simulink model "model_VS_PSH"  (R2020b)
settings: Solver=ode1  StartTime=0.0  StopTime=60  RelTol=1e-3
InitFcn:
  | xInitial = init_power_wind_dfig_det;
  | %Ts=5e-6;
values from neighbouring files (symbols this model uses):
  Cap_DClink = 20000e-6    (= 0.02)    [MAIN_VS_PSH.m]
  Efficiency = 0.9    [MAIN_VS_PSH.m]
  Fnom = 60    [MAIN_VS_PSH.m]
  H = 2.7    [MAIN_VS_PSH.m]
  Initial_Head = 1    [MAIN_VS_PSH.m]
  Initial_SOC = 0.8    [MAIN_VS_PSH.m]
  kmVdc = 20e3    (= 20000)    [MAIN_VS_PSH.m]
  Kp = 1    [MAIN_VS_PSH.m]
  kp_pll = 0.236583    [MAIN_T_PSH_IEEE39.m]    (also in MAIN_VS_PSH.m)
  Kpg = 1.3466e-5    (= 1.3466e-05)    [MAIN_VS_PSH.m]
  Kpr = 4.559e-5    (= 4.559e-05)    [MAIN_VS_PSH.m]
  Kvp = 6.1584    [MAIN_VS_PSH.m]
  Lm = Lb*Lmpu    [MAIN_VS_PSH.m]
  Lph = 3e-4    (= 0.0003)    [MAIN_VS_PSH.m]
  Lr = Lb*Lrpu    [MAIN_VS_PSH.m]
  Lrleakpu = 0.11    [MAIN_VS_PSH.m]
  Ls = Lb*Lspu    [MAIN_VS_PSH.m]
  Lsleakpu = 0.102    [MAIN_VS_PSH.m]
  Max_discharge_hrs = 10    [MAIN_VS_PSH.m]
  Mode = 0    [MAIN_FS_PSH_IEEE39.m]    (also in MAIN_VS_PSH.m = 1; plots_FS_PSH_IEEE39.m = 1; plots_VS_PSH.m = 1)
  Pnom = Srated*1e6    (= 300000000)    [MAIN_VS_PSH.m]
  Pref = 0.9    [MAIN_T_PSH_IEEE39.m]    (also in MAIN_VS_PSH.m = 1)
  QnL = 0    [MAIN_VS_PSH.m]
  Qref = 0    [MAIN_VS_PSH.m]
  Rrpu = 0.00607    [MAIN_VS_PSH.m]
  Rspu = 0.0054    [MAIN_VS_PSH.m]
  sigma = 1- Lmpu*Lmpu/(Lrpu^2)    (= 0.0485899542692)    [MAIN_VS_PSH.m]
  Srated = 300    [MAIN_VS_PSH.m]
  t_sw_off = 220    [MAIN_FS_PSH_IEEE39.m]    (also in MAIN_T_PSH_IEEE39.m; MAIN_VS_PSH.m = 45)
  t_sw_on = 130    [MAIN_FS_PSH_IEEE39.m]    (also in MAIN_T_PSH_IEEE39.m; MAIN_VS_PSH.m = 35)
  Ti = 0.01    [MAIN_VS_PSH.m]
  ti_pll = 0.0224242    [MAIN_T_PSH_IEEE39.m]    (also in MAIN_VS_PSH.m)
  Tig = 59.0944    [MAIN_VS_PSH.m]
  Tir = 197.953    [MAIN_VS_PSH.m]
  Ts = 25e-6    (= 2.5e-05)    [MAIN_FS_PSH_IEEE39.m]    (also in MAIN_T_PSH_IEEE39.m; MAIN_VS_PSH.m = 1e-07)
  TurnsRatio = 0.37912    [MAIN_VS_PSH.m]
  Tvi = 0.0013532    [MAIN_VS_PSH.m]
  V1 = sqrt(2)*Vnom_grid/sqrt(3)    [MAIN_VS_PSH.m]
  Vdc_ref = 40e3    (= 40000)    [MAIN_VS_PSH.m]
  Vnom_grid = 18e3    (= 18000)    [MAIN_VS_PSH.m]
  W1 = 2*pi*Fnom    (= 376.991118431)    [MAIN_VS_PSH.m]
  Xph = Lph*W1    (= 0.113097335529)    [MAIN_VS_PSH.m]
undefined symbols (not defined in the file or in its folder): magnitude
libraries: powerlib x49, powerlib_meascontrol x21, pid_lib x10, simulink_extras x4, simulink x1
(part 2 of 3)

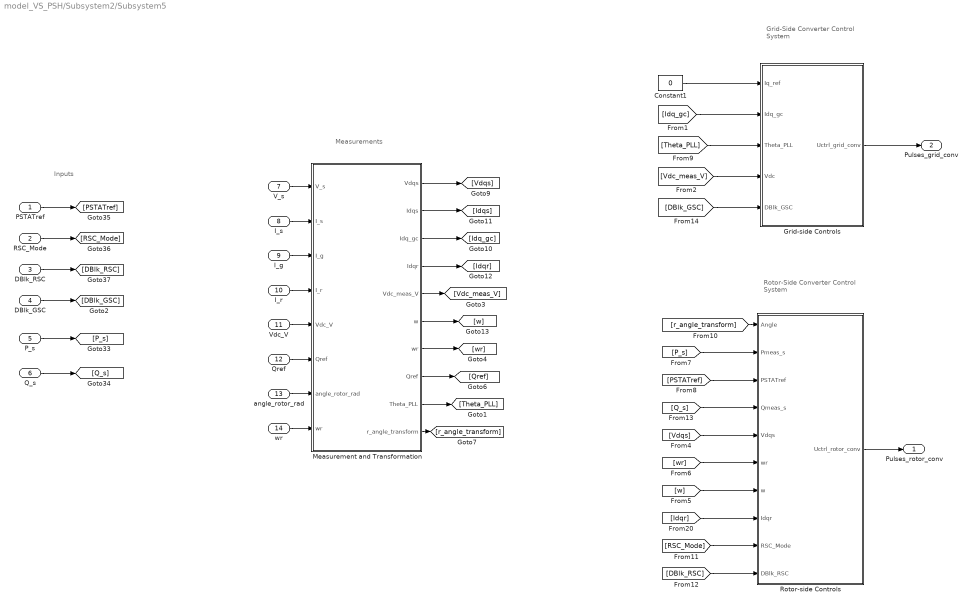
== system model_VS_PSH/Subsystem2/Subsystem5 ==
  note: Measurements
  note: Inputs
  note: Grid-Side Converter
      | Control System
  note: Rotor-Side Converter
      | Control System
  PSTATref : Inport
  RSC_Mode : Inport  Port=2
  DBlk_RSC : Inport  Port=3
  DBlk_GSC : Inport  Port=4
  P_s : Inport  Port=5
  Q_s : Inport  Port=6
  V_s : Inport  Port=7
  I_s : Inport  Port=8
  I_g : Inport  Port=9
  I_r : Inport  Port=10
  Vdc_V : Inport  Port=11
  Qref : Inport  Port=12
  angle_rotor_rad : Inport  Port=13
  wr : Inport  Port=14
  Constant1 : Constant  Value=0
  Grid-side Controls : Subsystem
  Measurement and Transformation : Subsystem
  Rotor-side Controls : Subsystem
  Pulses_rotor_conv : Outport  VectorParamsAs1DForOutWhenUnconnected=off
  Pulses_grid_conv : Outport  Port=2  VectorParamsAs1DForOutWhenUnconnected=off
  wires:
  PSTATref/1 -> [PSTATref]
  Q_s/1 -> [Q_s]
  P_s/1 -> [P_s]
  RSC_Mode/1 -> [RSC_Mode]
  DBlk_GSC/1 -> [DBlk_GSC]
  DBlk_RSC/1 -> [DBlk_RSC]
  Measurement and Transformation/7("wr ") -> [wr]
  Qref/1 -> Measurement and Transformation/6(Qref)
  wr/1 -> Measurement and Transformation/8(wr)
  Measurement and Transformation/5(Vdc_meas_V) -> [Vdc_meas_V]
  V_s/1 -> Measurement and Transformation/1(V_s)
  I_g/1 -> Measurement and Transformation/3(I_g)
  I_s/1 -> Measurement and Transformation/2(I_s)
  Measurement and Transformation/3(Idq_gc) -> [Idq_gc]
  Measurement and Transformation/4(Idqr) -> [Idqr]
  angle_rotor_rad/1 -> Measurement and Transformation/7(angle_rotor_rad)
  Measurement and Transformation/8("Qref ") -> [Qref]
  Measurement and Transformation/9(Theta_PLL) -> [Theta_PLL]
  Measurement and Transformation/1(Vdqs) -> [Vdqs]
  Measurement and Transformation/10(r_angle_transform) -> [r_angle_transform]
  Measurement and Transformation/2(Idqs) -> [Idqs]
  Measurement and Transformation/6(w) -> [w]
  Vdc_V/1 -> Measurement and Transformation/5(Vdc_V)
  I_r/1 -> Measurement and Transformation/4(I_r)
  Rotor-side Controls/1(Uctrl_rotor_conv) -> Pulses_rotor_conv/1
  [P_s] -> Rotor-side Controls/2(Pmeas_s)
  [DBlk_GSC] -> Grid-side Controls/5(DBlk_GSC)
  Grid-side Controls/1(Uctrl_grid_conv) -> Pulses_grid_conv/1
  [RSC_Mode] -> Rotor-side Controls/9(RSC_Mode)
  [PSTATref] -> Rotor-side Controls/3(PSTATref)
  [wr] -> Rotor-side Controls/6(wr)
  [DBlk_RSC] -> Rotor-side Controls/10(DBlk_RSC)
  [Idqr] -> Rotor-side Controls/8(Idqr)
  [r_angle_transform] -> Rotor-side Controls/1(Angle)
  [Idq_gc] -> Grid-side Controls/2(Idq_gc)
  [Vdqs] -> Rotor-side Controls/5(Vdqs)
  [Theta_PLL] -> Grid-side Controls/3(Theta_PLL)
  Constant1/1 -> Grid-side Controls/1(Iq_ref)
  [Q_s] -> Rotor-side Controls/4(Qmeas_s)
  [Vdc_meas_V] -> Grid-side Controls/4(Vdc)
  [w] -> Rotor-side Controls/7(w)

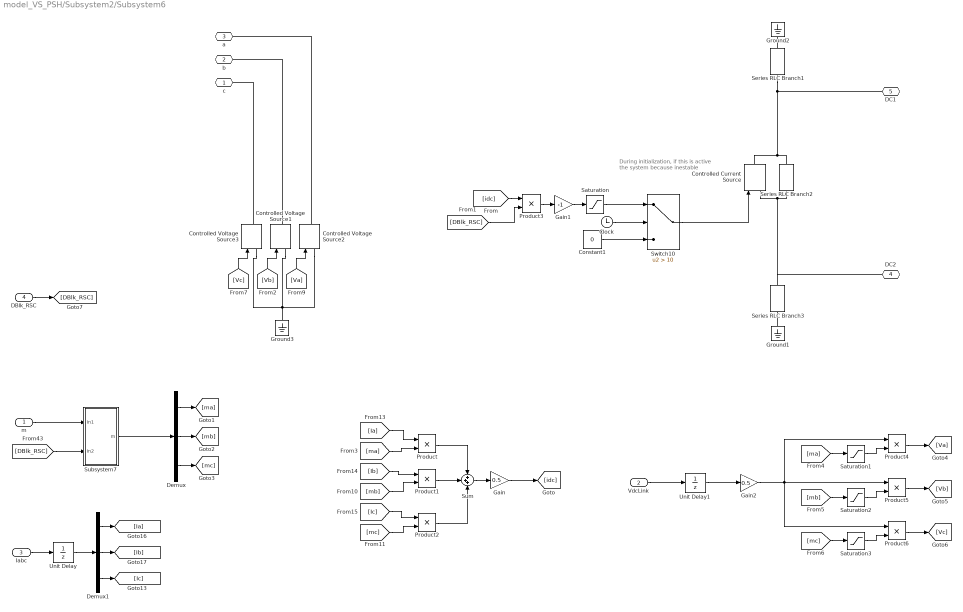
== system model_VS_PSH/Subsystem2/Subsystem6 ==
  note: During initialization, if this is active the system because inestable
  m : Inport
  VdcLink : Inport  Port=2
  Iabc : Inport  Port=3
  DBlk_RSC : Inport  Port=4
  Clock : Clock
  Constant1 : Constant  Value=0
  Controlled Current Source : powerlib/Electrical Sources/Controlled Current Source  Initialize=on  Source_Type=AC  Amplitude=0  Phase=0  Frequency=0  Measurements=None
  Controlled Voltage Source1 : powerlib/Electrical Sources/Controlled Voltage Source  Initialize=on  Source_Type=AC  Amplitude=0  Phase=0  Frequency=0  Measurements=None
  Controlled Voltage Source2 : powerlib/Electrical Sources/Controlled Voltage Source  Initialize=on  Source_Type=AC  Amplitude=0  Phase=0  Frequency=0  Measurements=None
  Controlled Voltage Source3 : powerlib/Electrical Sources/Controlled Voltage Source  Initialize=on  Source_Type=AC  Amplitude=0  Phase=0  Frequency=0  Measurements=None
  Demux : Demux  Outputs=3
  Demux1 : Demux  Outputs=3
  Gain : Gain  Gain=0.5
  Gain1 : Gain  Gain=-1
  Gain2 : Gain  Gain=0.5
  Ground1 : powerlib/Elements/Ground  LConnTagsString=a
  Ground2 : powerlib/Elements/Ground  LConnTagsString=a
  Ground3 : powerlib/Elements/Ground  LConnTagsString=a
  Product{,1..6} (7 alike) : Product
  Saturation : Saturate  UpperLimit=1e10  LowerLimit=-1e10
  Saturation1 : Saturate  UpperLimit=1  LowerLimit=-1
  Saturation2 : Saturate  UpperLimit=1  LowerLimit=-1
  Saturation3 : Saturate  UpperLimit=1  LowerLimit=-1
  Series RLC Branch1 : powerlib/Elements/Series RLC Branch  LConnTagsString=__new0  RConnTagsString=__new0  BranchType=R  Resistance=1e6  Inductance=1e-3  SetiL0=off  InitialCurrent=0  Capacitance=1e-6  Setx0=off  InitialVoltage=0  Measurements=None
  Series RLC Branch2 : powerlib/Elements/Series RLC Branch  LConnTagsString=__new0  RConnTagsString=__new0  BranchType=R  Resistance=1e6  Inductance=1e-3  SetiL0=off  InitialCurrent=0  Capacitance=1e-6  Setx0=off  InitialVoltage=0  Measurements=None
  Series RLC Branch3 : powerlib/Elements/Series RLC Branch  LConnTagsString=__new0  RConnTagsString=__new0  BranchType=R  Resistance=1e6  Inductance=1e-3  SetiL0=off  InitialCurrent=0  Capacitance=1e-6  Setx0=off  InitialVoltage=0  Measurements=None
  Subsystem7 : Subsystem
  Sum : Sum  Inputs=+++
  Switch10 : Switch  Criteria=u2 > Threshold  Threshold=10
  Unit Delay : UnitDelay  SampleTime=-1  HasFrameUpgradeWarning=on
  Unit Delay1 : UnitDelay  SampleTime=-1  HasFrameUpgradeWarning=on
  c : PMIOPort  Side=Left
  b : PMIOPort  Port=2  Side=Left
  a : PMIOPort  Port=3  Side=Left
  DC2 : PMIOPort  Port=4  Side=Right
  DC1 : PMIOPort  Port=5  Side=Right
  wires:
  [Vb] -> Controlled Voltage Source1/1
  [Va] -> Controlled Voltage Source2/1
  [Ib] -> Product1/1
  Product6/1 -> [Vc]
  [ma] -> Saturation1/1
  [DBlk_RSC] -> Product3/2
  [mc] -> Product2/2
  Product/1 -> Sum/1
  [Ic] -> Product2/1
  Product3/1 -> Gain1/1
  Saturation3/1 -> Product6/2
  [idc] -> Product3/1
  [Vc] -> Controlled Voltage Source3/1
  Saturation2/1 -> Product5/2
  [mb] -> Product1/2
  Product4/1 -> [Va]
  Gain1/1 -> Saturation/1
  [Ia] -> Product/1
  [mc] -> Saturation3/1
  Product1/1 -> Sum/2
  [mb] -> Saturation2/1
  Saturation1/1 -> Product4/2
  [ma] -> Product/2
  Product2/1 -> Sum/3
  Product5/1 -> [Vb]
  Gain2/1 -> Product4/1, Product5/1, Product6/1
  Gain/1 -> [idc]
  Sum/1 -> Gain/1
  Demux/1 -> [ma]
  Demux/2 -> [mb]
  Demux/3 -> [mc]
  Demux1/2 -> [Ib]
  Demux1/1 -> [Ia]
  Demux1/3 -> [Ic]
  m/1 -> Subsystem7/1(In1)
  [DBlk_RSC] -> Subsystem7/2(In2)
  Switch10/1 -> Controlled Current Source/1
  Saturation/1 -> Switch10/1
  Clock/1 -> Switch10/2
  Constant1/1 -> Switch10/3
  Subsystem7/1(m) -> Demux/1
  DBlk_RSC/1 -> [DBlk_RSC]
  VdcLink/1 -> Unit Delay1/1
  Unit Delay1/1 -> Gain2/1
  Iabc/1 -> Unit Delay/1
  Unit Delay/1 -> Demux1/1
  connections:
  Controlled Voltage Source2/RConn1 -- a/RConn1
  Controlled Voltage Source3/RConn1 -- c/RConn1
  DC1/RConn1 -- Series RLC Branch1/RConn1 -- Series RLC Branch2/LConn1 -- Controlled Current Source/RConn1
  Series RLC Branch3/LConn1 -- DC2/RConn1 -- Controlled Current Source/LConn1 -- Series RLC Branch2/RConn1
  Controlled Voltage Source1/LConn1 -- Ground3/LConn1 -- Controlled Voltage Source2/LConn1 -- Controlled Voltage Source3/LConn1
  Controlled Voltage Source1/RConn1 -- b/RConn1
  Ground1/LConn1 -- Series RLC Branch3/RConn1
  Series RLC Branch1/LConn1 -- Ground2/LConn1

== system model_VS_PSH/Subsystem2/Subsystem/PI Control Governor ==
  WTurErr : Inport
  RSC_mode : Inport  Port=2
  Constant2 : Constant  Value=0
  Integrator : Integrator  ExternalReset=rising  UpperSaturationLimit=100  LowerSaturationLimit=-100
  KpGov : Constant  Value=0.001
  Product4 : Product
  Product5 : Product
  Saturation3 : Saturate  UpperLimit=100  LowerLimit=-100
  Sum7 : Sum  Inputs=++|
  Switch8 : Switch  Criteria=u2 > Threshold
  TiGov : Constant  Value=0.01
  TurOut : Outport
  wires:
  KpGov/1 -> Product4/1
  Product4/1 -> Sum7/1
  Saturation3/1 -> Sum7/2
  Integrator/1 -> Saturation3/1
  TiGov/1 -> Product5/1
  Sum7/1 -> TurOut/1
  WTurErr/1 -> Product5/2, Product4/2
  Product5/1 -> Switch8/1
  Switch8/1 -> Integrator/1
  Constant2/1 -> Switch8/3
  RSC_mode/1 -> Integrator/2, Switch8/2

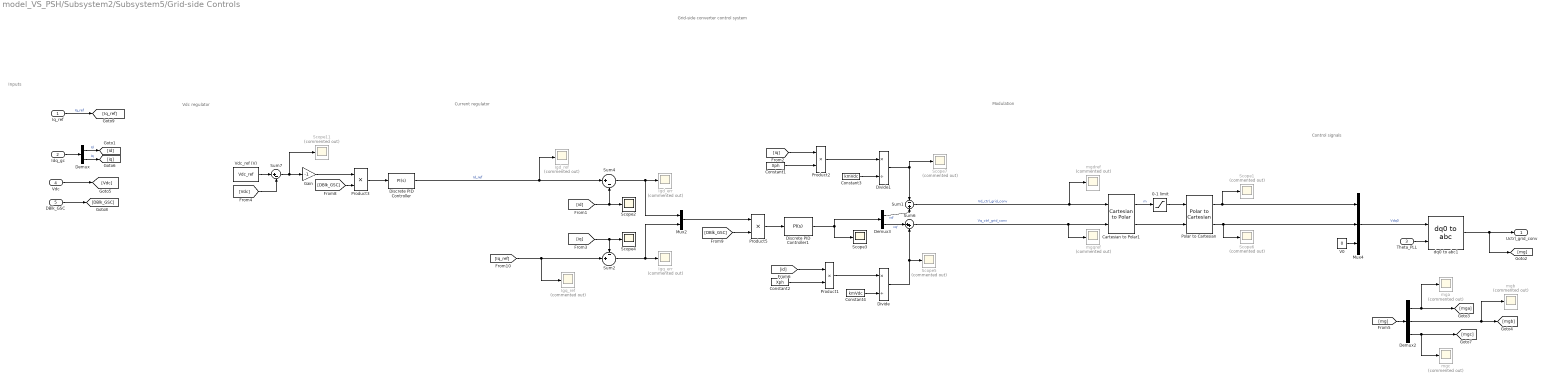
== system model_VS_PSH/Subsystem2/Subsystem5/Grid-side Controls ==
  note: Control signals
  note: Modulation
  note: Current regulator
  note: Vdc regulator
  note: Inputs
  note: Grid-side converter control system
  Iq_ref : Inport
  Idq_gc : Inport  Port=2
  Theta_PLL : Inport  Port=3
  Vdc : Inport  Port=4
  DBlk_GSC : Inport  Port=5
  0-1 limit : Saturate  UpperLimit=1  LowerLimit=0
  Cartesian to Polar1 : simulink_extras/Transformations/Cartesian to Polar
  Constant1 : Constant  Value=Xph
  Constant2 : Constant  Value=Xph
  Constant3 : Constant  Value=kmVdc
  Constant4 : Constant  Value=kmVdc
  Demux : Demux  Outputs=2
      settings: DisplayOption=none
  Demux2 : Demux  Outputs=3
      settings: DisplayOption=none
  Demux3 : Demux  Outputs=2
      settings: DisplayOption=none
  Discrete PID Controller : pid_lib/PID Controller  Controller=PI  Form=Parallel  TimeDomain=Continuous-time  UseExternalTs=off  SampleTime=-1  IntegratorMethod=Forward Euler  FilterMethod=Forward Euler  ControllerParametersSource=internal  P=Kvp  I=Kvp/Tvi  D=0  UseFilter=on  N=100  TunerSelectOption=Transfer Function Based (PID Tuner App)  InitialConditionSource=internal  InitialConditionForIntegrator=0  InitialConditionForFilter=0  DifferentiatorICPrevScaledInput=0  ExternalReset=none  TrackingMode=off  Kt=1  LimitOutput=off  SatLimitsSource=internal  UpperSaturationLimit=inf  LowerSaturationLimit=-inf  LinearizeAsGain=off  AntiWindupMode=none  Kb=1  POutMin=[]  POutMax=[]  IOutMin=[]  IOutMax=[]  DOutMin=[]  DOutMax=[]  NOutMin=[]  NOutMax=[]  SumOutMin=[]  SumOutMax=[]  SaturationOutMin=[]  SaturationOutMax=[]  PParamMin=[]  PParamMax=[]  IParamMin=[]  IParamMax=[]  DParamMin=[]  DParamMax=[]  NParamMin=[]  NParamMax=[]  KbParamMin=[]  KbParamMax=[]  KtParamMin=[]  KtParamMax=[]  KbOutMin=[]  KbOutMax=[]  KtOutMin=[]  KtOutMax=[]  IntegratorOutMin=[]  IntegratorOutMax=[]  FilterOutMin=[]  FilterOutMax=[]  SumI1OutMin=[]  SumI1OutMax=[]  SumI2OutMin=[]  SumI2OutMax=[]  SumI3OutMin=[]  SumI3OutMax=[]  SumI4OutMin=[]  SumI4OutMax=[]  SumDOutMin=[]  SumDOutMax=[]  DifferentiatorOutMin=[]  DifferentiatorOutMax=[]  FilterDiffOutCoefMin=[]  FilterDiffOutCoefMax=[]  ReciprocalOutMin=[]  ReciprocalOutMax=[]  SumDenOutMin=[]  SumDenOutMax=[]  SumNumOutMin=[]  SumNumOutMax=[]  DivideOutMin=[]  DivideOutMax=[]  UdiffTsProdOutMin=[]  UdiffTsProdOutMax=[]  NTsProdOutMin=[]  NTsProdOutMax=[]  UintegralTsProdOutMin=[]  UintegralTsProdOutMax=[]  UngainTsProdOutMin=[]  UngainTsProdOutMax=[]  IntegratorContinuousStateAttributes=''  IntegratorStateMustResolveToSignalObject=off  IntegratorRTWStateStorageClass=Auto  FilterContinuousStateAttributes=''  FilterStateMustResolveToSignalObject=off  FilterRTWStateStorageClass=Auto  ParallelPVariant=InternalParameters  IdealPVariant=Disabled  IVariant=InternalParameters  DVariant=Disabled  IntegratorVariant=Continuous  SatVariant=Disabled  AWVariant=Passthrough  PCopyVariant=Disabled  TRVariant=Disabled  FdbkBlocksVariant=Forward  IdealPFdbkVariant=Disabled  SatFdbkVariant=Disabled  DerivativeFilterVariant=Disabled  NVariant=Disabled  NCopyVariant=Disabled_SignalSpec  FilterICVariant=Disabled  IntegratorICVariant=InternalICs  ExternalResetVariant=Disabled  TRSumVariant=Passthrough  SumFdbkVariant=Disabled  SumVariant=Sum_PI  TsampFilterVariant=InternalTs  TsampNgainVariant=Passthrough  TsampIntegralVariant=Passthrough  ExternalSaturationOutDataTypeStr=Inherit: Same as second input
  Discrete PID Controller1 : pid_lib/PID Controller  Controller=PI  Form=Parallel  TimeDomain=Continuous-time  UseExternalTs=off  SampleTime=-1  IntegratorMethod=Forward Euler  FilterMethod=Forward Euler  ControllerParametersSource=internal  P=Kpg  I=Kpg/Tig  D=0  UseFilter=on  N=100  TunerSelectOption=Transfer Function Based (PID Tuner App)  InitialConditionSource=internal  InitialConditionForIntegrator=0  InitialConditionForFilter=0  DifferentiatorICPrevScaledInput=0  ExternalReset=none  TrackingMode=off  Kt=1  LimitOutput=off  SatLimitsSource=internal  UpperSaturationLimit=inf  LowerSaturationLimit=-inf  LinearizeAsGain=off  AntiWindupMode=none  Kb=1  POutMin=[]  POutMax=[]  IOutMin=[]  IOutMax=[]  DOutMin=[]  DOutMax=[]  NOutMin=[]  NOutMax=[]  SumOutMin=[]  SumOutMax=[]  SaturationOutMin=[]  SaturationOutMax=[]  PParamMin=[]  PParamMax=[]  IParamMin=[]  IParamMax=[]  DParamMin=[]  DParamMax=[]  NParamMin=[]  NParamMax=[]  KbParamMin=[]  KbParamMax=[]  KtParamMin=[]  KtParamMax=[]  KbOutMin=[]  KbOutMax=[]  KtOutMin=[]  KtOutMax=[]  IntegratorOutMin=[]  IntegratorOutMax=[]  FilterOutMin=[]  FilterOutMax=[]  SumI1OutMin=[]  SumI1OutMax=[]  SumI2OutMin=[]  SumI2OutMax=[]  SumI3OutMin=[]  SumI3OutMax=[]  SumI4OutMin=[]  SumI4OutMax=[]  SumDOutMin=[]  SumDOutMax=[]  DifferentiatorOutMin=[]  DifferentiatorOutMax=[]  FilterDiffOutCoefMin=[]  FilterDiffOutCoefMax=[]  ReciprocalOutMin=[]  ReciprocalOutMax=[]  SumDenOutMin=[]  SumDenOutMax=[]  SumNumOutMin=[]  SumNumOutMax=[]  DivideOutMin=[]  DivideOutMax=[]  UdiffTsProdOutMin=[]  UdiffTsProdOutMax=[]  NTsProdOutMin=[]  NTsProdOutMax=[]  UintegralTsProdOutMin=[]  UintegralTsProdOutMax=[]  UngainTsProdOutMin=[]  UngainTsProdOutMax=[]  IntegratorContinuousStateAttributes=''  IntegratorStateMustResolveToSignalObject=off  IntegratorRTWStateStorageClass=Auto  FilterContinuousStateAttributes=''  FilterStateMustResolveToSignalObject=off  FilterRTWStateStorageClass=Auto  ParallelPVariant=InternalParameters  IdealPVariant=Disabled  IVariant=InternalParameters  DVariant=Disabled  IntegratorVariant=Continuous  SatVariant=Disabled  AWVariant=Passthrough  PCopyVariant=Disabled  TRVariant=Disabled  FdbkBlocksVariant=Forward  IdealPFdbkVariant=Disabled  SatFdbkVariant=Disabled  DerivativeFilterVariant=Disabled  NVariant=Disabled  NCopyVariant=Disabled_SignalSpec  FilterICVariant=Disabled  IntegratorICVariant=InternalICs  ExternalResetVariant=Disabled  TRSumVariant=Passthrough  SumFdbkVariant=Disabled  SumVariant=Sum_PI  TsampFilterVariant=InternalTs  TsampNgainVariant=Passthrough  TsampIntegralVariant=Passthrough  ExternalSaturationOutDataTypeStr=Inherit: Same as second input
  Divide : Product  Inputs=*/
  Divide1 : Product  Inputs=*/
  Gain : Gain  Gain=-1
  Igd_err : Scope  Commented=on
  Igd_ref : Scope  Commented=on
  Igq_err : Scope  Commented=on
  Igq_ref : Scope  Commented=on
  Mux2 : Mux  Inputs=2
  Mux4 : Mux  Inputs=3
  Polar to Cartesian : simulink_extras/Transformations/Polar to Cartesian
      settings: SourceProductBaseCode=SL
  Product1 : Product  InputSameDT=on  SaturateOnIntegerOverflow=on  OutDataTypeStr=Inherit: Same as first input
  Product2 : Product  InputSameDT=on  SaturateOnIntegerOverflow=on  OutDataTypeStr=Inherit: Same as first input
  Product3 : Product
  Product5 : Product
  Scope{1,5..7,11} (5 alike) : Scope  Commented=on
  Scope2 : Scope
  Scope3 : Scope
  Scope4 : Scope
  Sum1 : Sum  Inputs=-+  InputSameDT=on  SaturateOnIntegerOverflow=on  OutDataTypeStr=Inherit: Same as first input
  Sum2 : Sum  Inputs=-+|  InputSameDT=on  SaturateOnIntegerOverflow=on  OutDataTypeStr=Inherit: Same as first input
  Sum4 : Sum  Inputs=|+-  InputSameDT=on  SaturateOnIntegerOverflow=on  OutDataTypeStr=Inherit: Same as first input
  Sum6 : Sum  Inputs=|++  InputSameDT=on  SaturateOnIntegerOverflow=on  OutDataTypeStr=Inherit: Same as first input
  Sum7 : Sum  Inputs=|+-  InputSameDT=on  SaturateOnIntegerOverflow=on  OutDataTypeStr=Inherit: Same as first input
  V0 : Constant  Value=0
  Vdc_ref (V) : Constant  Value=Vdc_ref
  dq0 to abc1 : powerlib_meascontrol/Transformations/dq0 to abc  Alignment=Aligned with phase A axis
  mga : Scope  Commented=on
  mgb : Scope  Commented=on
  mgc : Scope  Commented=on
  mgdref : Scope  Commented=on
  mgqref : Scope  Commented=on
  Uctrl_grid_conv : Outport  VectorParamsAs1DForOutWhenUnconnected=off
  wires:
  Sum6/1 -> mgqref/1, Cartesian to Polar1/2  "Vq_ctrl_grid_conv"
  Sum1/1 -> mgdref/1, Cartesian to Polar1/1  "Vd_ctrl_grid_conv"
  Mux4/1 -> dq0 to abc1/1  "Vdq0"
  Polar to Cartesian/2 -> Scope6/1, Mux4/2
  Polar to Cartesian/1 -> Scope1/1, Mux4/1
  V0/1 -> Mux4/3
  Cartesian to Polar1/1 -> 0-1 limit/1  "m"
  0-1 limit/1 -> Polar to Cartesian/1
  Cartesian to Polar1/2 -> Polar to Cartesian/2
  Idq_gc/1 -> Demux/1
  Constant2/1 -> Product1/2
  Discrete PID Controller1/1 -> Demux3/1, Scope3/1
  Sum4/1 -> Mux2/1, Igd_err/1
  Sum2/1 -> Igq_err/1, Mux2/2
  Demux3/1 -> Sum1/2  "vd'"
  Demux3/2 -> Sum6/1  "vq'"
  Discrete PID Controller/1 -> Sum4/1, Igd_ref/1  "Id_ref"
  Vdc_ref (V)/1 -> Sum7/1
  Demux/1 -> [id]  "Id"
  Demux/2 -> [iq]  "Iq"
  Product1/1 -> Divide/1
  Constant4/1 -> Divide/2
  Divide/1 -> Scope5/1, Sum6/2
  Product2/1 -> Divide1/1
  Constant1/1 -> Product2/2
  Constant3/1 -> Divide1/2
  Divide1/1 -> Scope7/1, Sum1/1
  Vdc/1 -> [Vdc]
  [Vdc] -> Sum7/2
  [iq] -> Scope4/1, Sum2/1
  [id] -> Scope2/1, Sum4/2
  [iq] -> Product2/1
  [id] -> Product1/1
  Demux2/2 -> mgb/1, [mgb]
  Demux2/1 -> mga/1, [mga]
  Demux2/3 -> [mgc], mgc/1
  [mg] -> Demux2/1
  [DBlk_GSC] -> Product3/2
  Product3/1 -> Discrete PID Controller/1
  Sum7/1 -> Gain/1, Scope11/1
  [DBlk_GSC] -> Product5/2
  Mux2/1 -> Product5/1
  Product5/1 -> Discrete PID Controller1/1
  DBlk_GSC/1 -> [DBlk_GSC]
  dq0 to abc1/1 -> Uctrl_grid_conv/1, [mg]
  Theta_PLL/1 -> dq0 to abc1/2
  Iq_ref/1 -> [Iq_ref]  "Iq_ref"
  [Iq_ref] -> Sum2/2, Igq_ref/1
  Gain/1 -> Product3/1

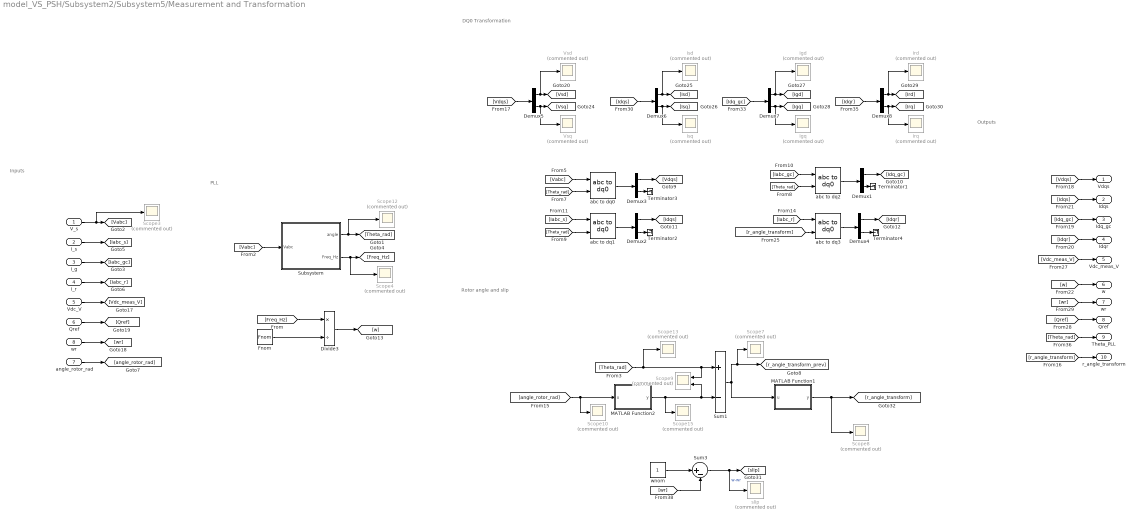
== system model_VS_PSH/Subsystem2/Subsystem5/Measurement and Transformation ==
  note: Outputs
  note: DQ0 Transformation
  note: Rotor angle and slip
  note: PLL
  note: Inputs
  V_s : Inport
  I_s : Inport  Port=2
  I_g : Inport  Port=3
  I_r : Inport  Port=4
  Vdc_V : Inport  Port=5
  Qref : Inport  Port=6
  angle_rotor_rad : Inport  Port=7
  wr : Inport  Port=8
  Demux{1..4} (4 alike) : Demux  Outputs=[2 1]
      settings: DisplayOption=none
  Demux{5..8} (4 alike) : Demux  Outputs=[1 1]
      settings: DisplayOption=none
  Divide3 : Product  Inputs=*/
  Fnom : Constant  Value=Fnom
  Igd : Scope  Commented=on
  Igq : Scope  Commented=on
  Ird : Scope  Commented=on
  Irq : Scope  Commented=on
  Isd : Scope  Commented=on
  Isq : Scope  Commented=on
  MATLAB Function1 : MATLAB Function  TreatAsAtomicUnit=on
  MATLAB Function2 : MATLAB Function  TreatAsAtomicUnit=on
  Scope{3..4,7..8,10,12..13,15} (8 alike) : Scope  Commented=on
  Scope9 : Scope  Commented=on  NumInputPorts=2
  Subsystem : Subsystem
  Sum1 : Sum  Inputs=+-  InputSameDT=on  SaturateOnIntegerOverflow=on  OutDataTypeStr=Inherit: Same as first input
  Sum3 : Sum  Inputs=|+-  InputSameDT=on  SaturateOnIntegerOverflow=on  OutDataTypeStr=Inherit: Same as first input
  Terminator{1..4} (4 alike) : Terminator
  Vsd : Scope  Commented=on
  Vsq : Scope  Commented=on
  abc to dq{0..3} (4 alike) : powerlib_meascontrol/Transformations/abc to dq0  Alignment=Aligned with phase A axis
  slip : Scope  Commented=on
  wnom : Constant
  Vdqs : Outport  VectorParamsAs1DForOutWhenUnconnected=off
  Idqs : Outport  Port=2  VectorParamsAs1DForOutWhenUnconnected=off
  Idq_gc : Outport  Port=3  VectorParamsAs1DForOutWhenUnconnected=off
  Idqr : Outport  Port=4  VectorParamsAs1DForOutWhenUnconnected=off
  Vdc_meas_V : Outport  Port=5  VectorParamsAs1DForOutWhenUnconnected=off
  w : Outport  Port=6  VectorParamsAs1DForOutWhenUnconnected=off
  "wr " : Outport  Port=7  VectorParamsAs1DForOutWhenUnconnected=off
  "Qref " : Outport  Port=8  VectorParamsAs1DForOutWhenUnconnected=off
  Theta_PLL : Outport  Port=9  VectorParamsAs1DForOutWhenUnconnected=off
  r_angle_transform : Outport  Port=10  VectorParamsAs1DForOutWhenUnconnected=off
  wires:
  [Vabc] -> Subsystem/1(Vabc)
  [r_angle_transform] -> r_angle_transform/1
  [Theta_rad] -> Theta_PLL/1
  Demux1/2 -> Terminator1/1
  Demux3/1 -> [Vdqs]
  Demux3/2 -> Terminator3/1
  abc to dq2/1 -> Demux1/1
  abc to dq0/1 -> Demux3/1
  Demux2/2 -> Terminator2/1
  abc to dq1/1 -> Demux2/1
  Fnom/1 -> Divide3/2
  Divide3/1 -> [w]
  [Freq_Hz] -> Divide3/1
  [Vabc] -> abc to dq0/1
  [Theta_rad] -> abc to dq0/2
  [Theta_rad] -> abc to dq2/2
  [Theta_rad] -> abc to dq1/2
  [Iabc_gc] -> abc to dq2/1
  [Iabc_s] -> abc to dq1/1
  [Iabc_r] -> abc to dq3/1
  Demux1/1 -> [Idq_gc]
  Demux2/1 -> [Idqs]
  [Vdqs] -> Vdqs/1
  [Idq_gc] -> Idq_gc/1
  [Idqr] -> Idqr/1
  [Idqs] -> Idqs/1
  [w] -> w/1
  [r_angle_transform] -> abc to dq3/2
  [Vdc_meas_V] -> Vdc_meas_V/1
  [Qref] -> "Qref "/1
  [wr] -> "wr "/1
  V_s/1 -> Scope3/1, [Vabc]
  I_s/1 -> [Iabc_s]
  I_g/1 -> [Iabc_gc]
  I_r/1 -> [Iabc_r]
  Vdc_V/1 -> [Vdc_meas_V]
  Qref/1 -> [Qref]
  wr/1 -> [wr]
  angle_rotor_rad/1 -> [angle_rotor_rad]
  [Theta_rad] -> Scope13/1, Sum1/1, Scope9/1
  [Vdqs] -> Demux5/1
  Demux5/1 -> Vsd/1, [Vsd]
  Demux5/2 -> Vsq/1, [Vsq]
  Demux6/2 -> Isq/1, [Isq]
  [Idqs] -> Demux6/1
  Demux6/1 -> Isd/1, [Isd]
  Demux7/2 -> Igq/1, [Igq]
  [Idq_gc] -> Demux7/1
  Demux7/1 -> Igd/1, [Igd]
  Demux8/2 -> Irq/1, [Irq]
  [Idqr] -> Demux8/1
  Demux8/1 -> Ird/1, [Ird]
  [wr] -> Sum3/2
  Sum3/1 -> slip/1, [slip]  "w-wr"
  Sum1/1 -> Scope7/1, [r_angle_transform_prev], MATLAB Function1/1(u)
  MATLAB Function1/1(y) -> Scope8/1, [r_angle_transform]
  abc to dq3/1 -> Demux4/1
  Demux4/1 -> [Idqr]
  Demux4/2 -> Terminator4/1
  wnom/1 -> Sum3/1
  Subsystem/2(Freq_Hz) -> [Freq_Hz], Scope4/1
  [angle_rotor_rad] -> Scope10/1, MATLAB Function2/1(u)
  Subsystem/1(angle) -> Scope12/1, [Theta_rad]
  MATLAB Function2/1(y) -> Scope15/1, Sum1/2, Scope9/2

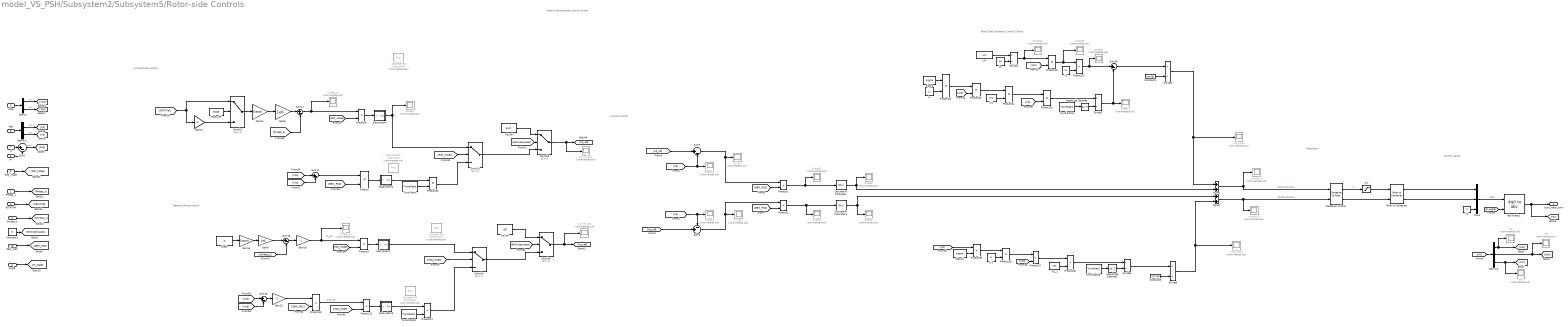
== system model_VS_PSH/Subsystem2/Subsystem5/Rotor-side Controls ==
  note: Control signals
  note: Modulation
  note: Current control
  note: Reactive Power control
  note: Active Power control
  note: Rotor-side converter control system
  note: Q_err
  note: Amp_err
  note: Rotor Side Converter Current Control
  Angle : Inport
  Pmeas_s : Inport  Port=2
  PSTATref : Inport  Port=3
  Qmeas_s : Inport  Port=4
  Vdqs : Inport  Port=5
  wr : Inport  Port=6
  w : Inport  Port=7
  Idqr : Inport  Port=8
  RSC_Mode : Inport  Port=9
  DBlk_RSC : Inport  Port=10
  0-1 : Saturate  UpperLimit=1  LowerLimit=0
  Cartesian to Polar : simulink_extras/Transformations/Cartesian to Polar
  Constant1 : Constant  Value=kmVdc
  Constant2 : Constant  Value=0
  Constant3 : Constant  Value=kmVdc
  Demux : Demux  Outputs=2
      settings: DisplayOption=none
  Demux1 : Demux  Outputs=2
      settings: DisplayOption=none
  Demux2 : Demux  Outputs=3
      settings: DisplayOption=none
  Discrete PI Controller : pid_lib/PID Controller  Controller=PI  Form=Parallel  TimeDomain=Continuous-time  UseExternalTs=off  SampleTime=-1  IntegratorMethod=Forward Euler  FilterMethod=Forward Euler  ControllerParametersSource=internal  P=Kpr  I=Kpr/Tir  D=0  UseFilter=on  N=100  TunerSelectOption=Transfer Function Based (PID Tuner App)  InitialConditionSource=internal  InitialConditionForIntegrator=0  InitialConditionForFilter=0  DifferentiatorICPrevScaledInput=0  ExternalReset=none  TrackingMode=off  Kt=1  LimitOutput=off  SatLimitsSource=internal  UpperSaturationLimit=inf  LowerSaturationLimit=-inf  LinearizeAsGain=off  AntiWindupMode=none  Kb=1  POutMin=[]  POutMax=[]  IOutMin=[]  IOutMax=[]  DOutMin=[]  DOutMax=[]  NOutMin=[]  NOutMax=[]  SumOutMin=[]  SumOutMax=[]  SaturationOutMin=[]  SaturationOutMax=[]  PParamMin=[]  PParamMax=[]  IParamMin=[]  IParamMax=[]  DParamMin=[]  DParamMax=[]  NParamMin=[]  NParamMax=[]  KbParamMin=[]  KbParamMax=[]  KtParamMin=[]  KtParamMax=[]  KbOutMin=[]  KbOutMax=[]  KtOutMin=[]  KtOutMax=[]  IntegratorOutMin=[]  IntegratorOutMax=[]  FilterOutMin=[]  FilterOutMax=[]  SumI1OutMin=[]  SumI1OutMax=[]  SumI2OutMin=[]  SumI2OutMax=[]  SumI3OutMin=[]  SumI3OutMax=[]  SumI4OutMin=[]  SumI4OutMax=[]  SumDOutMin=[]  SumDOutMax=[]  DifferentiatorOutMin=[]  DifferentiatorOutMax=[]  FilterDiffOutCoefMin=[]  FilterDiffOutCoefMax=[]  ReciprocalOutMin=[]  ReciprocalOutMax=[]  SumDenOutMin=[]  SumDenOutMax=[]  SumNumOutMin=[]  SumNumOutMax=[]  DivideOutMin=[]  DivideOutMax=[]  UdiffTsProdOutMin=[]  UdiffTsProdOutMax=[]  NTsProdOutMin=[]  NTsProdOutMax=[]  UintegralTsProdOutMin=[]  UintegralTsProdOutMax=[]  UngainTsProdOutMin=[]  UngainTsProdOutMax=[]  IntegratorContinuousStateAttributes=''  IntegratorStateMustResolveToSignalObject=off  IntegratorRTWStateStorageClass=Auto  FilterContinuousStateAttributes=''  FilterStateMustResolveToSignalObject=off  FilterRTWStateStorageClass=Auto  ParallelPVariant=InternalParameters  IdealPVariant=Disabled  IVariant=InternalParameters  DVariant=Disabled  IntegratorVariant=Continuous  SatVariant=Disabled  AWVariant=Passthrough  PCopyVariant=Disabled  TRVariant=Disabled  FdbkBlocksVariant=Forward  IdealPFdbkVariant=Disabled  SatFdbkVariant=Disabled  DerivativeFilterVariant=Disabled  NVariant=Disabled  NCopyVariant=Disabled_SignalSpec  FilterICVariant=Disabled  IntegratorICVariant=InternalICs  ExternalResetVariant=Disabled  TRSumVariant=Passthrough  SumFdbkVariant=Disabled  SumVariant=Sum_PI  TsampFilterVariant=InternalTs  TsampNgainVariant=Passthrough  TsampIntegralVariant=Passthrough  ExternalSaturationOutDataTypeStr=Inherit: Same as second input
  Discrete PI Controller1 : pid_lib/PID Controller  Controller=PI  Form=Parallel  TimeDomain=Continuous-time  UseExternalTs=off  SampleTime=-1  IntegratorMethod=Forward Euler  FilterMethod=Forward Euler  ControllerParametersSource=internal  P=Kpr  I=Kpr/Tir  D=0  UseFilter=on  N=100  TunerSelectOption=Transfer Function Based (PID Tuner App)  InitialConditionSource=internal  InitialConditionForIntegrator=0  InitialConditionForFilter=0  DifferentiatorICPrevScaledInput=0  ExternalReset=none  TrackingMode=off  Kt=1  LimitOutput=off  SatLimitsSource=internal  UpperSaturationLimit=inf  LowerSaturationLimit=-inf  LinearizeAsGain=off  AntiWindupMode=none  Kb=1  POutMin=[]  POutMax=[]  IOutMin=[]  IOutMax=[]  DOutMin=[]  DOutMax=[]  NOutMin=[]  NOutMax=[]  SumOutMin=[]  SumOutMax=[]  SaturationOutMin=[]  SaturationOutMax=[]  PParamMin=[]  PParamMax=[]  IParamMin=[]  IParamMax=[]  DParamMin=[]  DParamMax=[]  NParamMin=[]  NParamMax=[]  KbParamMin=[]  KbParamMax=[]  KtParamMin=[]  KtParamMax=[]  KbOutMin=[]  KbOutMax=[]  KtOutMin=[]  KtOutMax=[]  IntegratorOutMin=[]  IntegratorOutMax=[]  FilterOutMin=[]  FilterOutMax=[]  SumI1OutMin=[]  SumI1OutMax=[]  SumI2OutMin=[]  SumI2OutMax=[]  SumI3OutMin=[]  SumI3OutMax=[]  SumI4OutMin=[]  SumI4OutMax=[]  SumDOutMin=[]  SumDOutMax=[]  DifferentiatorOutMin=[]  DifferentiatorOutMax=[]  FilterDiffOutCoefMin=[]  FilterDiffOutCoefMax=[]  ReciprocalOutMin=[]  ReciprocalOutMax=[]  SumDenOutMin=[]  SumDenOutMax=[]  SumNumOutMin=[]  SumNumOutMax=[]  DivideOutMin=[]  DivideOutMax=[]  UdiffTsProdOutMin=[]  UdiffTsProdOutMax=[]  NTsProdOutMin=[]  NTsProdOutMax=[]  UintegralTsProdOutMin=[]  UintegralTsProdOutMax=[]  UngainTsProdOutMin=[]  UngainTsProdOutMax=[]  IntegratorContinuousStateAttributes=''  IntegratorStateMustResolveToSignalObject=off  IntegratorRTWStateStorageClass=Auto  FilterContinuousStateAttributes=''  FilterStateMustResolveToSignalObject=off  FilterRTWStateStorageClass=Auto  ParallelPVariant=InternalParameters  IdealPVariant=Disabled  IVariant=InternalParameters  DVariant=Disabled  IntegratorVariant=Continuous  SatVariant=Disabled  AWVariant=Passthrough  PCopyVariant=Disabled  TRVariant=Disabled  FdbkBlocksVariant=Forward  IdealPFdbkVariant=Disabled  SatFdbkVariant=Disabled  DerivativeFilterVariant=Disabled  NVariant=Disabled  NCopyVariant=Disabled_SignalSpec  FilterICVariant=Disabled  IntegratorICVariant=InternalICs  ExternalResetVariant=Disabled  TRSumVariant=Passthrough  SumFdbkVariant=Disabled  SumVariant=Sum_PI  TsampFilterVariant=InternalTs  TsampNgainVariant=Passthrough  TsampIntegralVariant=Passthrough  ExternalSaturationOutDataTypeStr=Inherit: Same as second input
  Discrete PID Controller1 : pid_lib/PID Controller  Commented=on  Controller=PI  Form=Parallel  TimeDomain=Continuous-time  UseExternalTs=off  SampleTime=-1  IntegratorMethod=Forward Euler  FilterMethod=Forward Euler  ControllerParametersSource=internal  P=Kp  I=Kp/Ti  D=0  UseFilter=on  N=100  TunerSelectOption=Transfer Function Based (PID Tuner App)  InitialConditionSource=internal  InitialConditionForIntegrator=0  InitialConditionForFilter=0  DifferentiatorICPrevScaledInput=0  ExternalReset=none  TrackingMode=off  Kt=1  LimitOutput=on  SatLimitsSource=internal  UpperSaturationLimit=10e3  LowerSaturationLimit=-10e3  LinearizeAsGain=off  AntiWindupMode=back-calculation  Kb=1  POutMin=[]  POutMax=[]  IOutMin=[]  IOutMax=[]  DOutMin=[]  DOutMax=[]  NOutMin=[]  NOutMax=[]  SumOutMin=[]  SumOutMax=[]  SaturationOutMin=[]  SaturationOutMax=[]  PParamMin=[]  PParamMax=[]  IParamMin=[]  IParamMax=[]  DParamMin=[]  DParamMax=[]  NParamMin=[]  NParamMax=[]  KbParamMin=[]  KbParamMax=[]  KtParamMin=[]  KtParamMax=[]  KbOutMin=[]  KbOutMax=[]  KtOutMin=[]  KtOutMax=[]  IntegratorOutMin=[]  IntegratorOutMax=[]  FilterOutMin=[]  FilterOutMax=[]  SumI1OutMin=[]  SumI1OutMax=[]  SumI2OutMin=[]  SumI2OutMax=[]  SumI3OutMin=[]  SumI3OutMax=[]  SumI4OutMin=[]  SumI4OutMax=[]  SumDOutMin=[]  SumDOutMax=[]  DifferentiatorOutMin=[]  DifferentiatorOutMax=[]  FilterDiffOutCoefMin=[]  FilterDiffOutCoefMax=[]  ReciprocalOutMin=[]  ReciprocalOutMax=[]  SumDenOutMin=[]  SumDenOutMax=[]  SumNumOutMin=[]  SumNumOutMax=[]  DivideOutMin=[]  DivideOutMax=[]  UdiffTsProdOutMin=[]  UdiffTsProdOutMax=[]  NTsProdOutMin=[]  NTsProdOutMax=[]  UintegralTsProdOutMin=[]  UintegralTsProdOutMax=[]  UngainTsProdOutMin=[]  UngainTsProdOutMax=[]  IntegratorContinuousStateAttributes=''  IntegratorStateMustResolveToSignalObject=off  IntegratorRTWStateStorageClass=Auto  FilterContinuousStateAttributes=''  FilterStateMustResolveToSignalObject=off  FilterRTWStateStorageClass=Auto  ParallelPVariant=InternalParameters  IdealPVariant=Disabled  IVariant=InternalParameters  DVariant=Disabled  IntegratorVariant=Continuous  SatVariant=Enabled  AWVariant=BackCalculation  PCopyVariant=Disabled  TRVariant=Disabled  FdbkBlocksVariant=Forward  IdealPFdbkVariant=Disabled  SatFdbkVariant=Disabled  DerivativeFilterVariant=Disabled  NVariant=Disabled  NCopyVariant=Disabled_SignalSpec  FilterICVariant=Disabled  IntegratorICVariant=InternalICs  ExternalResetVariant=Disabled  TRSumVariant=Passthrough  SumFdbkVariant=Disabled  SumVariant=Sum_PI  TsampFilterVariant=InternalTs  TsampNgainVariant=Passthrough  TsampIntegralVariant=Passthrough  ExternalSaturationOutDataTypeStr=Inherit: Same as second input
  Discrete PID Controller2 : pid_lib/PID Controller  Commented=on  Controller=PI  Form=Parallel  TimeDomain=Continuous-time  UseExternalTs=off  SampleTime=-1  IntegratorMethod=Forward Euler  FilterMethod=Forward Euler  ControllerParametersSource=internal  P=Kp  I=Kp/Ti  D=0  UseFilter=on  N=100  TunerSelectOption=Transfer Function Based (PID Tuner App)  InitialConditionSource=internal  InitialConditionForIntegrator=0  InitialConditionForFilter=0  DifferentiatorICPrevScaledInput=0  ExternalReset=none  TrackingMode=off  Kt=1  LimitOutput=on  SatLimitsSource=internal  UpperSaturationLimit=10e3  LowerSaturationLimit=-10e3  LinearizeAsGain=off  AntiWindupMode=back-calculation  Kb=1  POutMin=[]  POutMax=[]  IOutMin=[]  IOutMax=[]  DOutMin=[]  DOutMax=[]  NOutMin=[]  NOutMax=[]  SumOutMin=[]  SumOutMax=[]  SaturationOutMin=[]  SaturationOutMax=[]  PParamMin=[]  PParamMax=[]  IParamMin=[]  IParamMax=[]  DParamMin=[]  DParamMax=[]  NParamMin=[]  NParamMax=[]  KbParamMin=[]  KbParamMax=[]  KtParamMin=[]  KtParamMax=[]  KbOutMin=[]  KbOutMax=[]  KtOutMin=[]  KtOutMax=[]  IntegratorOutMin=[]  IntegratorOutMax=[]  FilterOutMin=[]  FilterOutMax=[]  SumI1OutMin=[]  SumI1OutMax=[]  SumI2OutMin=[]  SumI2OutMax=[]  SumI3OutMin=[]  SumI3OutMax=[]  SumI4OutMin=[]  SumI4OutMax=[]  SumDOutMin=[]  SumDOutMax=[]  DifferentiatorOutMin=[]  DifferentiatorOutMax=[]  FilterDiffOutCoefMin=[]  FilterDiffOutCoefMax=[]  ReciprocalOutMin=[]  ReciprocalOutMax=[]  SumDenOutMin=[]  SumDenOutMax=[]  SumNumOutMin=[]  SumNumOutMax=[]  DivideOutMin=[]  DivideOutMax=[]  UdiffTsProdOutMin=[]  UdiffTsProdOutMax=[]  NTsProdOutMin=[]  NTsProdOutMax=[]  UintegralTsProdOutMin=[]  UintegralTsProdOutMax=[]  UngainTsProdOutMin=[]  UngainTsProdOutMax=[]  IntegratorContinuousStateAttributes=''  IntegratorStateMustResolveToSignalObject=off  IntegratorRTWStateStorageClass=Auto  FilterContinuousStateAttributes=''  FilterStateMustResolveToSignalObject=off  FilterRTWStateStorageClass=Auto  ParallelPVariant=InternalParameters  IdealPVariant=Disabled  IVariant=InternalParameters  DVariant=Disabled  IntegratorVariant=Continuous  SatVariant=Enabled  AWVariant=BackCalculation  PCopyVariant=Disabled  TRVariant=Disabled  FdbkBlocksVariant=Forward  IdealPFdbkVariant=Disabled  SatFdbkVariant=Disabled  DerivativeFilterVariant=Disabled  NVariant=Disabled  NCopyVariant=Disabled_SignalSpec  FilterICVariant=Disabled  IntegratorICVariant=InternalICs  ExternalResetVariant=Disabled  TRSumVariant=Passthrough  SumFdbkVariant=Disabled  SumVariant=Sum_PI  TsampFilterVariant=InternalTs  TsampNgainVariant=Passthrough  TsampIntegralVariant=Passthrough  ExternalSaturationOutDataTypeStr=Inherit: Same as second input
  Discrete PID Controller3 : pid_lib/PID Controller  Commented=on  Controller=PI  Form=Parallel  TimeDomain=Continuous-time  UseExternalTs=off  SampleTime=-1  IntegratorMethod=Forward Euler  FilterMethod=Forward Euler  ControllerParametersSource=internal  P=Kp  I=Kp/Ti  D=0  UseFilter=on  N=100  TunerSelectOption=Transfer Function Based (PID Tuner App)  InitialConditionSource=internal  InitialConditionForIntegrator=0  InitialConditionForFilter=0  DifferentiatorICPrevScaledInput=0  ExternalReset=none  TrackingMode=off  Kt=1  LimitOutput=on  SatLimitsSource=internal  UpperSaturationLimit=10e3  LowerSaturationLimit=-10e3  LinearizeAsGain=off  AntiWindupMode=back-calculation  Kb=1  POutMin=[]  POutMax=[]  IOutMin=[]  IOutMax=[]  DOutMin=[]  DOutMax=[]  NOutMin=[]  NOutMax=[]  SumOutMin=[]  SumOutMax=[]  SaturationOutMin=[]  SaturationOutMax=[]  PParamMin=[]  PParamMax=[]  IParamMin=[]  IParamMax=[]  DParamMin=[]  DParamMax=[]  NParamMin=[]  NParamMax=[]  KbParamMin=[]  KbParamMax=[]  KtParamMin=[]  KtParamMax=[]  KbOutMin=[]  KbOutMax=[]  KtOutMin=[]  KtOutMax=[]  IntegratorOutMin=[]  IntegratorOutMax=[]  FilterOutMin=[]  FilterOutMax=[]  SumI1OutMin=[]  SumI1OutMax=[]  SumI2OutMin=[]  SumI2OutMax=[]  SumI3OutMin=[]  SumI3OutMax=[]  SumI4OutMin=[]  SumI4OutMax=[]  SumDOutMin=[]  SumDOutMax=[]  DifferentiatorOutMin=[]  DifferentiatorOutMax=[]  FilterDiffOutCoefMin=[]  FilterDiffOutCoefMax=[]  ReciprocalOutMin=[]  ReciprocalOutMax=[]  SumDenOutMin=[]  SumDenOutMax=[]  SumNumOutMin=[]  SumNumOutMax=[]  DivideOutMin=[]  DivideOutMax=[]  UdiffTsProdOutMin=[]  UdiffTsProdOutMax=[]  NTsProdOutMin=[]  NTsProdOutMax=[]  UintegralTsProdOutMin=[]  UintegralTsProdOutMax=[]  UngainTsProdOutMin=[]  UngainTsProdOutMax=[]  IntegratorContinuousStateAttributes=''  IntegratorStateMustResolveToSignalObject=off  IntegratorRTWStateStorageClass=Auto  FilterContinuousStateAttributes=''  FilterStateMustResolveToSignalObject=off  FilterRTWStateStorageClass=Auto  ParallelPVariant=InternalParameters  IdealPVariant=Disabled  IVariant=InternalParameters  DVariant=Disabled  IntegratorVariant=Continuous  SatVariant=Enabled  AWVariant=BackCalculation  PCopyVariant=Disabled  TRVariant=Disabled  FdbkBlocksVariant=Forward  IdealPFdbkVariant=Disabled  SatFdbkVariant=Disabled  DerivativeFilterVariant=Disabled  NVariant=Disabled  NCopyVariant=Disabled_SignalSpec  FilterICVariant=Disabled  IntegratorICVariant=InternalICs  ExternalResetVariant=Disabled  TRSumVariant=Passthrough  SumFdbkVariant=Disabled  SumVariant=Sum_PI  TsampFilterVariant=InternalTs  TsampNgainVariant=Passthrough  TsampIntegralVariant=Passthrough  ExternalSaturationOutDataTypeStr=Inherit: Same as second input
  Discrete PID Controller4 : pid_lib/PID Controller  Commented=on  Controller=PI  Form=Parallel  TimeDomain=Continuous-time  UseExternalTs=off  SampleTime=-1  IntegratorMethod=Forward Euler  FilterMethod=Forward Euler  ControllerParametersSource=internal  P=Kp  I=Kp/Ti  D=0  UseFilter=on  N=100  TunerSelectOption=Transfer Function Based (PID Tuner App)  InitialConditionSource=internal  InitialConditionForIntegrator=0  InitialConditionForFilter=0  DifferentiatorICPrevScaledInput=0  ExternalReset=none  TrackingMode=off  Kt=1  LimitOutput=on  SatLimitsSource=internal  UpperSaturationLimit=100e3  LowerSaturationLimit=-100e3  LinearizeAsGain=off  AntiWindupMode=back-calculation  Kb=1  POutMin=[]  POutMax=[]  IOutMin=[]  IOutMax=[]  DOutMin=[]  DOutMax=[]  NOutMin=[]  NOutMax=[]  SumOutMin=[]  SumOutMax=[]  SaturationOutMin=[]  SaturationOutMax=[]  PParamMin=[]  PParamMax=[]  IParamMin=[]  IParamMax=[]  DParamMin=[]  DParamMax=[]  NParamMin=[]  NParamMax=[]  KbParamMin=[]  KbParamMax=[]  KtParamMin=[]  KtParamMax=[]  KbOutMin=[]  KbOutMax=[]  KtOutMin=[]  KtOutMax=[]  IntegratorOutMin=[]  IntegratorOutMax=[]  FilterOutMin=[]  FilterOutMax=[]  SumI1OutMin=[]  SumI1OutMax=[]  SumI2OutMin=[]  SumI2OutMax=[]  SumI3OutMin=[]  SumI3OutMax=[]  SumI4OutMin=[]  SumI4OutMax=[]  SumDOutMin=[]  SumDOutMax=[]  DifferentiatorOutMin=[]  DifferentiatorOutMax=[]  FilterDiffOutCoefMin=[]  FilterDiffOutCoefMax=[]  ReciprocalOutMin=[]  ReciprocalOutMax=[]  SumDenOutMin=[]  SumDenOutMax=[]  SumNumOutMin=[]  SumNumOutMax=[]  DivideOutMin=[]  DivideOutMax=[]  UdiffTsProdOutMin=[]  UdiffTsProdOutMax=[]  NTsProdOutMin=[]  NTsProdOutMax=[]  UintegralTsProdOutMin=[]  UintegralTsProdOutMax=[]  UngainTsProdOutMin=[]  UngainTsProdOutMax=[]  IntegratorContinuousStateAttributes=''  IntegratorStateMustResolveToSignalObject=off  IntegratorRTWStateStorageClass=Auto  FilterContinuousStateAttributes=''  FilterStateMustResolveToSignalObject=off  FilterRTWStateStorageClass=Auto  ParallelPVariant=InternalParameters  IdealPVariant=Disabled  IVariant=InternalParameters  DVariant=Disabled  IntegratorVariant=Continuous  SatVariant=Enabled  AWVariant=BackCalculation  PCopyVariant=Disabled  TRVariant=Disabled  FdbkBlocksVariant=Forward  IdealPFdbkVariant=Disabled  SatFdbkVariant=Disabled  DerivativeFilterVariant=Disabled  NVariant=Disabled  NCopyVariant=Disabled_SignalSpec  FilterICVariant=Disabled  IntegratorICVariant=InternalICs  ExternalResetVariant=Disabled  TRSumVariant=Passthrough  SumFdbkVariant=Disabled  SumVariant=Sum_PI  TsampFilterVariant=InternalTs  TsampNgainVariant=Passthrough  TsampIntegralVariant=Passthrough  ExternalSaturationOutDataTypeStr=Inherit: Same as second input
  Divide{1..5} (5 alike) : Product  Inputs=*/
  Gain13 : Gain  Gain=-1
  Gain14 : Gain  Gain=Srated
  Gain16 : Gain  Gain=Srated
  Gain18 : Gain  Gain=-1
  Gain19 : Gain  Gain=-1
  Gain8 : Gain  Gain=1e6
  Gain9 : Gain  Gain=1e6
  Ird_err : Scope  Commented=on
  Ird_ref : Constant  Value=1147
  Ird_ref_plot : Scope  Commented=on
  Irq_err : Scope  Commented=on
  Irq_ref : Constant  Value=-257
  Irq_ref_plot : Scope  Commented=on
  Lm : Constant  Value=Lm
  Lr : Constant  Value=Lr
  Lr1 : Constant  Value=Lr
  Ls : Constant  Value=Ls
  Magnitude Squared : Math  Operator=magnitude^2  SaturateOnIntegerOverflow=on
  Magnitude Squared1 : Math  Operator=magnitude^2  SaturateOnIntegerOverflow=on
  Mode_del : Constant  Value=Mode  VectorParams1D=off
  Mux4 : Mux  Inputs=3
  P_dfig_err : Scope  Commented=on
  Polar to Cartesian : simulink_extras/Transformations/Polar to Cartesian
      settings: SourceProductBaseCode=SL
  Product{,1..2,8..12,15,19,22..30} (19 alike) : Product
  Q_dfig_err : Scope  Commented=on
  Qref1 : Constant  Value=0
  Scope{1..7,15..16,18..19} (11 alike) : Scope  Commented=on
  Subsystem1 : Subsystem
  Subsystem2 : Subsystem
  Subsystem3 : Subsystem
  Subsystem4 : Subsystem
  Sum1 : Sum  Inputs=|+-  InputSameDT=on  SaturateOnIntegerOverflow=on  OutDataTypeStr=Inherit: Same as first input
  Sum{14,17..20} (5 alike) : Sum  Inputs=|+-
  Sum4 : Sum  Inputs=-+|  InputSameDT=on  SaturateOnIntegerOverflow=on  OutDataTypeStr=Inherit: Same as first input
  Sum5 : Sum  Inputs=|+-  InputSameDT=on  SaturateOnIntegerOverflow=on  OutDataTypeStr=Inherit: Same as first input
  Sum6 : Sum  InputSameDT=on  SaturateOnIntegerOverflow=on  OutDataTypeStr=Inherit: Same as first input
  Sum8 : Sum  InputSameDT=on  SaturateOnIntegerOverflow=on  OutDataTypeStr=Inherit: Same as first input
  Switch{1..2,4..6} (5 alike) : Switch  Criteria=u2 > Threshold
  Turnd Ratio1 : Constant  Value=TurnsRatio
  Turnd Ratio2 : Constant  Value=TurnsRatio
  Turnd Ratio3 : Constant  Value=TurnsRatio
  Turns Ratio : Constant  Value=TurnsRatio
  V0 : Constant  Value=0
  V1 : Constant  Value=V1
  Vrd_comp : Scope  Commented=on
  Vrq_comp : Scope  Commented=on
  W1 : Constant  Value=W1
  W1_2 : Constant  Value=W1
  dq0 to abc1 : powerlib_meascontrol/Transformations/dq0 to abc  Alignment=Aligned with phase A axis
  mar : Scope  Commented=on
  mbr : Scope  Commented=on
  mcr : Scope  Commented=on
  rcontrol_d : Scope  Commented=on
  rcontrol_q : Scope  Commented=on
  sigma : Constant  Value=sigma
  sigma1 : Constant  Value=sigma
  Uctrl_rotor_conv : Outport  VectorParamsAs1DForOutWhenUnconnected=off
  wires:
  0-1/1 -> Polar to Cartesian/1
  Polar to Cartesian/2 -> Mux4/2
  Polar to Cartesian/1 -> Mux4/1
  Cartesian to Polar/2 -> Polar to Cartesian/2
  Cartesian to Polar/1 -> 0-1/1  "m"
  Sum8/1 -> rcontrol_q/1, Cartesian to Polar/2  "Vq_ctrl_rotor_conv"
  Sum6/1 -> rcontrol_d/1, Cartesian to Polar/1  "Vd_ctrl_rotor_conv"
  Mux4/1 -> dq0 to abc1/1  "Vdq0"
  V0/1 -> Mux4/3
  Product11/1 -> Switch4/3
  [Vsd] -> Sum19/2
  [Vsq] -> Sum17/2
  Sum18/1 -> Gain18/1
  Qref1/1 -> Gain16/1
  Switch2/1 -> Gain14/1
  Switch6/1 -> Irq_ref_plot/1, [Irq_ref]
  [BlkOuterLoops] -> Switch6/2
  Turns Ratio/1 -> Product10/2
  [RSC_Mode] -> Switch1/2
  Switch5/1 -> Ird_ref_plot/1, [Ird_ref]
  Subsystem2/1(Out) -> Switch4/1
  [Qmeas_s] -> Sum18/2
  Subsystem3/1(Out) -> Product11/1
  Turnd Ratio3/1 -> Product11/2
  Ird_ref/1 -> Switch5/1
  [PSTATref] -> Switch2/1, Gain13/1
  Product10/1 -> Switch1/3
  Switch4/1 -> Switch6/3
  [RSC_Mode] -> Switch4/2
  Gain19/1 -> Product19/1
  [Pmeas_s] -> Sum14/2
  [BlkOuterLoops] -> Switch5/2
  Sum17/1 -> Product/1
  Subsystem1/1(Out) -> Product10/1
  Sum19/1 -> Gain19/1
  Mode_del/1 -> Switch2/2
  [DBlk_RSC] -> Product19/2
  Irq_ref/1 -> Switch6/1
  Switch1/1 -> Switch5/3
  [Vsq] -> Sum17/1
  [DBlk_RSC] -> Product/2
  [Vsd] -> Sum19/1
  Gain13/1 -> Switch2/3
  Qmeas_s/1 -> [Qmeas_s]
  RSC_Mode/1 -> [RSC_Mode]
  PSTATref/1 -> [PSTATref]
  Pmeas_s/1 -> [Pmeas_s]
  Demux/2 -> [Vsq]  "Iq"
  Demux/1 -> [Vsd]  "Id"
  w/1 -> Sum1/1
  Vdqs/1 -> Demux/1
  Sum1/1 -> [slip]  "w-wr"
  wr/1 -> Sum1/2
  Constant2/1 -> [BlkOuterLoops]
  W1/1 -> Product24/2
  Product26/1 -> Divide2/1
  Ls/1 -> Divide1/2
  Product15/1 -> Product22/1, Scope19/1
  Magnitude Squared/1 -> Divide2/2
  Product25/1 -> Product23/1
  Divide2/1 -> Sum20/2, Scope7/1
  Product23/1 -> Product24/1
  V1/1 -> Product22/2
  [slip] -> Product15/2
  Lm/1 -> Divide1/1
  Divide1/1 -> Product15/1, Scope18/1
  [slip] -> Product23/2
  Lr/1 -> Product25/2
  Product24/1 -> Product26/1
  Turnd Ratio1/1 -> Magnitude Squared/1
  sigma/1 -> Product25/1
  Product22/1 -> Sum20/1, Scope6/1
  Product30/1 -> Product29/1
  W1_2/1 -> Product28/2
  Product29/1 -> Product27/1
  [slip] -> Product27/2
  sigma1/1 -> Product30/2
  Product27/1 -> Product28/1
  Lr1/1 -> Product29/2
  Magnitude Squared1/1 -> Divide5/2
  Product28/1 -> Divide5/1
  Turnd Ratio2/1 -> Magnitude Squared1/1
  Idqr/1 -> Demux1/1
  Demux1/2 -> [Irq]  "Iqr"
  Demux1/1 -> [Ird]  "Idr"
  [Irq] -> Product26/2
  [Ird] -> Product30/1
  [Irq_ref] -> Sum4/2
  [Ird] -> Sum5/2, Scope16/1
  [Irq] -> Sum4/1, Scope3/1
  Demux2/2 -> mbr/1, [mbr]
  Demux2/3 -> mcr/1, [mcr]
  Demux2/1 -> mar/1, [mar]
  [mr] -> Demux2/1
  [RSC_Mode] -> Product8/2
  Sum14/1 -> Product8/1, P_dfig_err/1
  Subsystem4/1(Out) -> Scope1/1, Switch1/1
  DBlk_RSC/1 -> [DBlk_RSC]
  Sum5/1 -> Product1/1, Ird_err/1
  Discrete PI Controller/1 -> Scope2/1, Sum6/2
  [DBlk_RSC] -> Product1/2
  Product1/1 -> Scope15/1, Discrete PI Controller/1
  Product2/1 -> Scope4/1, Discrete PI Controller1/1
  [DBlk_RSC] -> Product2/2
  Sum4/1 -> Product2/1, Irq_err/1
  Discrete PI Controller1/1 -> Scope5/1, Sum8/1
  [Ird_ref] -> Sum5/1
  Product8/1 -> Subsystem4/1(In)
  Product/1 -> Subsystem1/1(In)
  Product9/1 -> Subsystem2/1(In)
  Gain18/1 -> Q_dfig_err/1, Product9/1
  [RSC_Mode] -> Product9/2
  Product12/1 -> Subsystem3/1(In)
  Product19/1 -> Product12/1
  [RSC_Mode] -> Product12/2
  Gain14/1 -> Gain8/1
  Gain8/1 -> Sum14/1
  Gain16/1 -> Gain9/1
  Gain9/1 -> Sum18/1
  dq0 to abc1/1 -> [mr], Uctrl_rotor_conv/1
  Angle/1 -> [R_angle]
  [R_angle] -> dq0 to abc1/2
  Divide3/1 -> Sum8/2, Vrq_comp/1
  Divide5/1 -> Divide3/1
  Constant3/1 -> Divide3/2
  Constant1/1 -> Divide4/2
  Sum20/1 -> Divide4/1
  Divide4/1 -> Vrd_comp/1, Sum6/1

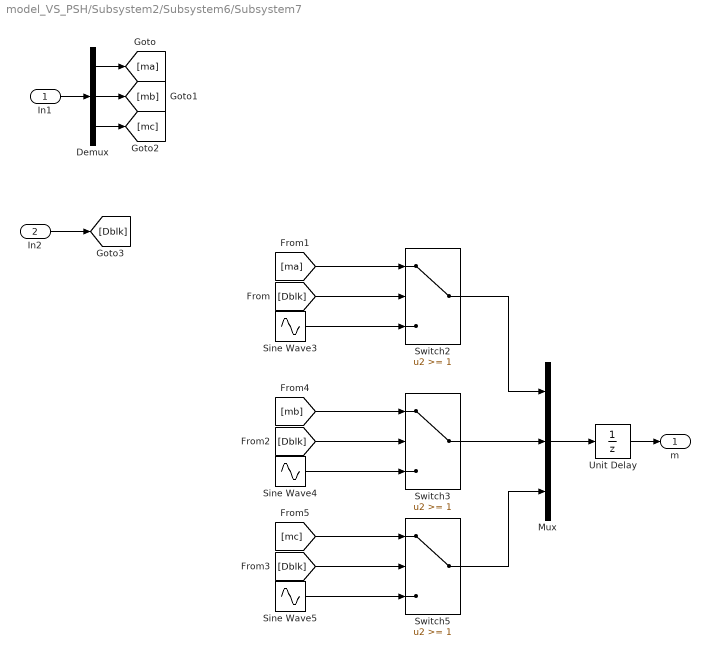
== system model_VS_PSH/Subsystem2/Subsystem6/Subsystem7 ==
  In1 : Inport
  In2 : Inport  Port=2
  Demux : Demux  Outputs=3
  Mux : Mux  Inputs=3
  Sine Wave3 : Sin  Amplitude=0  Frequency=376.99  SampleTime=0
  Sine Wave4 : Sin  Amplitude=0  Frequency=376.99  Phase=-120*pi/180  SampleTime=0
  Sine Wave5 : Sin  Amplitude=0  Frequency=376.99  Phase=120*pi/180  SampleTime=0
  Switch2 : Switch  Threshold=1
  Switch3 : Switch  Threshold=1
  Switch5 : Switch  Threshold=1
  Unit Delay : UnitDelay  SampleTime=-1  HasFrameUpgradeWarning=on
  m : Outport
  wires:
  In1/1 -> Demux/1
  Demux/1 -> [ma]
  Demux/2 -> [mb]
  Demux/3 -> [mc]
  In2/1 -> [Dblk]
  [Dblk] -> Switch2/2
  [Dblk] -> Switch3/2
  [Dblk] -> Switch5/2
  [ma] -> Switch2/1
  [mb] -> Switch3/1
  [mc] -> Switch5/1
  Sine Wave3/1 -> Switch2/3
  Sine Wave4/1 -> Switch3/3
  Switch3/1 -> Mux/2
  Switch2/1 -> Mux/1
  Sine Wave5/1 -> Switch5/3
  Switch5/1 -> Mux/3
  Unit Delay/1 -> m/1
  Mux/1 -> Unit Delay/1
